simulink model "two"  (R2014a)
settings: Solver=ode3  StartTime=0.0  StopTime=30  FixedStep=0.1  RelTol=1e-3
libraries: simulink x6
settings Model: Creator=Павел  LastModifiedBy=Павел
settings DataIOCC: InspectSignalLogs=on

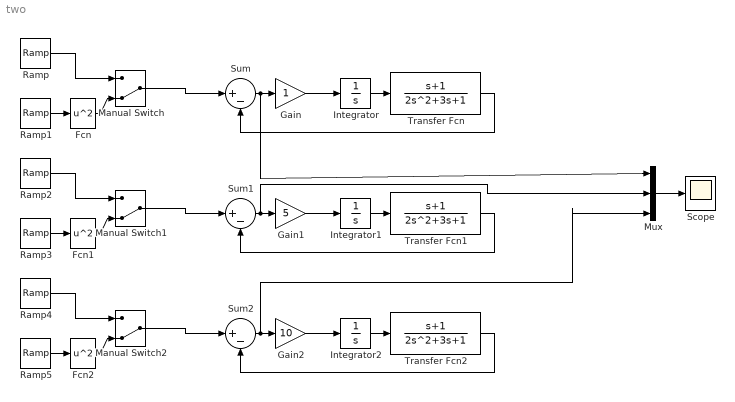
== system two ==
  Fcn : Fcn  Expr=u^2
  Fcn1 : Fcn  Expr=u^2
  Fcn2 : Fcn  Expr=u^2
  Gain : Gain
  Gain1 : Gain  Gain=5
  Gain2 : Gain  Gain=10
  Integrator : Integrator
  Integrator1 : Integrator
  Integrator2 : Integrator
  Manual Switch : ManualSwitch  CurrentSetting=0
  Manual Switch1 : ManualSwitch  CurrentSetting=0
  Manual Switch2 : ManualSwitch  CurrentSetting=0
  Mux : Mux  Inputs=3
  Ramp : simulink/Sources/Ramp  slope=1.5  start=0  X0=0
  Ramp1 : simulink/Sources/Ramp  slope=0.5  start=0  X0=0
  Ramp2 : simulink/Sources/Ramp  slope=1.5  start=0  X0=0
  Ramp3 : simulink/Sources/Ramp  slope=0.5  start=0  X0=0
  Ramp4 : simulink/Sources/Ramp  slope=1.5  start=0  X0=0
  Ramp5 : simulink/Sources/Ramp  slope=0.25  start=0  X0=0
  Scope : Scope
      settings: TimeRange=30
  Sum : Sum  Inputs=|+-
  Sum1 : Sum  Inputs=|+-
  Sum2 : Sum  Inputs=|+-
  Transfer Fcn : TransferFcn  Numerator=[1 1]  Denominator=[2 3 1]
  Transfer Fcn1 : TransferFcn  Numerator=[1 1]  Denominator=[2 3 1]
  Transfer Fcn2 : TransferFcn  Numerator=[1 1]  Denominator=[2 3 1]
  wires:
  Sum/1 -> Mux/1, Gain/1
  Gain/1 -> Integrator/1
  Integrator/1 -> Transfer Fcn/1
  Ramp/1 -> Manual Switch/1
  Ramp1/1 -> Fcn/1
  Fcn/1 -> Manual Switch/2
  Transfer Fcn/1 -> Sum/2
  Sum1/1 -> Mux/2, Gain1/1
  Gain1/1 -> Integrator1/1
  Integrator1/1 -> Transfer Fcn1/1
  Ramp2/1 -> Manual Switch1/1
  Ramp3/1 -> Fcn1/1
  Fcn1/1 -> Manual Switch1/2
  Transfer Fcn1/1 -> Sum1/2
  Sum2/1 -> Mux/3, Gain2/1
  Gain2/1 -> Integrator2/1
  Integrator2/1 -> Transfer Fcn2/1
  Ramp4/1 -> Manual Switch2/1
  Ramp5/1 -> Fcn2/1
  Fcn2/1 -> Manual Switch2/2
  Transfer Fcn2/1 -> Sum2/2
  Mux/1 -> Scope/1
  Manual Switch/1 -> Sum/1
  Manual Switch1/1 -> Sum1/1
  Manual Switch2/1 -> Sum2/1
